simulink model "Charge_2_V1"  (R2017b)
settings: Solver=FixedStepDiscrete  StartTime=0.0  StopTime=1  FixedStep=0.001  RelTol=1e-3
PreLoadFcn:
  | librarySetup
  | eval([bdroot,'_startup']) %Calling [modelName]_startup.m
undefined symbols (not defined in the file or in its folder): A0, A1, Car1__Authorize, Car2_Authorize, CON2, CON3, CON4, Control_Mode_In, CurrentSP, D10, D12, D13, D2, D3, D4, D5, D6, D7, D8, Frequency_High_Point, Frequency_Low_Point, Frequency_Mid_high, Frequency_Mid_low, HVol_High_Point, HVol_Low_Point, HVol_Mid_high, HVol_Mid_low, HVoltage_Factor, SeconCar_ThreePhase, V_Current_five, V_Current_four, V_Current_one, V_Current_six, V_Current_three, V_Current_two, V_Frequency, V_MaxPliot, V_MinPliot, Vol_High_Point, Vol_Low_Point, Vol_Mid_high, Vol_Mid_low, Voltage_Factor, Voltage_Mode_Test
libraries: simulink x331, HANcoder_STM32_Target x30, powerlib_meascontrol x8, simulink_extras x2
(part 2 of 13)

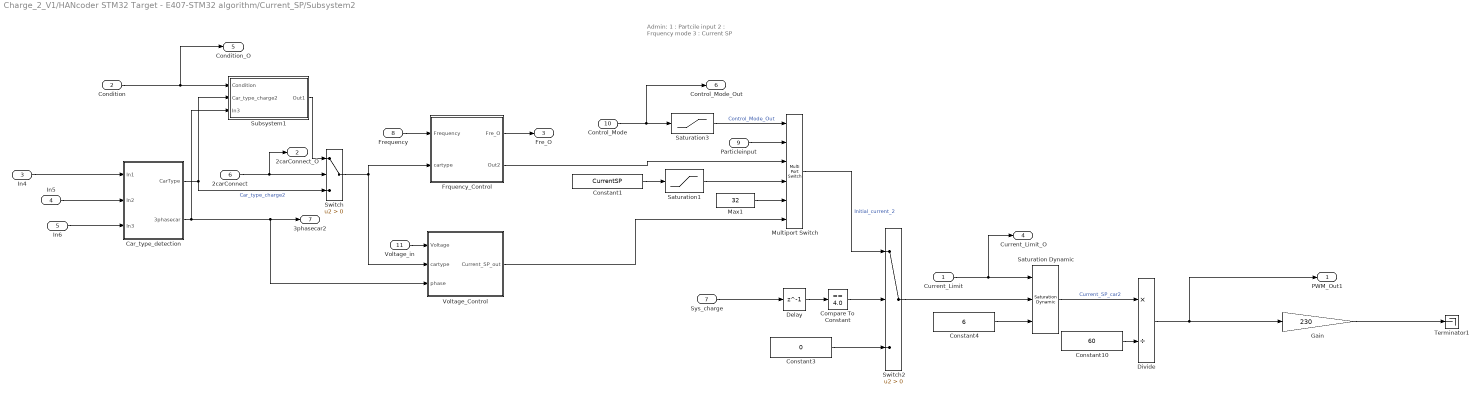
== system Charge_2_V1/HANcoder STM32 Target - E407-STM32 algorithm/Current_SP/Subsystem2 ==
  note: Admin:   1 : Partcile input
      | 		2 : Frquency mode
      | 		3 : Current SP
  Current_Limit : Inport
  Condition : Inport  Port=2
  In4 : Inport  Port=3
  In5 : Inport  Port=4
  In6 : Inport  Port=5
  2carConnect : Inport  Port=6
  Sys_charge : Inport  Port=7
  Frequency : Inport  Port=8
  Particleinput : Inport  Port=9
  Control_Mode : Inport  Port=10
  Voltage_in : Inport  Port=11
  Car_type_detection : Subsystem
  Compare To Constant : simulink/Logic and Bit Operations/Compare To Constant  relop===  const=4.0  OutDataTypeStr=boolean
  Constant1 : Constant  Value=CurrentSP  OutDataTypeStr=single  SampleTime=-1
  Constant10 : Constant  Value=60  OutDataTypeStr=single  SampleTime=-1
  Constant3 : Constant  Value=0  OutDataTypeStr=single  SampleTime=-1
  Constant4 : Constant  Value=6  OutDataTypeStr=single  SampleTime=-1
  Delay : Delay  DelayLength=1  InitialCondition=0
  Divide : Product  Inputs=*/
  Frquency_Control : Subsystem
  Gain : Gain  Gain=230  OutDataTypeStr=single
  Max1 : Constant  Value=32  OutDataTypeStr=single  SampleTime=-1
  Multiport Switch : MultiPortSwitch  Inputs=5
  Saturation Dynamic : simulink/Discontinuities/Saturation Dynamic  OutMin=[]  OutMax=[]  OutDataTypeStr=Inherit: Same as second input  OutDataType=fixdt(1, 16)  OutScaling=2^-10  DoSatur=off
  Saturation1 : Saturate  UpperLimit=32  LowerLimit=6
  Saturation3 : Saturate  UpperLimit=5  LowerLimit=1
  Subsystem1 : Subsystem
  Switch : Switch  Criteria=u2 > Threshold
  Switch2 : Switch  Criteria=u2 > Threshold
  Terminator1 : Terminator
  Voltage_Control : Subsystem
  PWM_Out1 : Outport
  2carConnect_O : Outport  Port=2
  Fre_O : Outport  Port=3
  Current_Limit_O : Outport  Port=4
  Condition_O : Outport  Port=5
  Control_Mode_Out : Outport  Port=6
  3phasecar2 : Outport  Port=7
  wires:
  Compare To Constant/1 -> Switch2/2
  Constant3/1 -> Switch2/3
  Delay/1 -> Compare To Constant/1
  Sys_charge/1 -> Delay/1
  Constant10/1 -> Divide/2
  In5/1 -> Car_type_detection/2(In2)
  Multiport Switch/1 -> Switch2/1  "Initial_current_2"
  In6/1 -> Car_type_detection/3(In3)
  In4/1 -> Car_type_detection/1(In1)
  Constant1/1 -> Saturation1/1
  Car_type_detection/1(CarType) -> Subsystem1/2(Car_type_charge2), Switch/3  "Car_type_charge2"
  Gain/1 -> Terminator1/1
  Divide/1 -> PWM_Out1/1, Gain/1
  Saturation1/1 -> Multiport Switch/4
  Switch2/1 -> Saturation Dynamic/2
  Constant4/1 -> Saturation Dynamic/3
  Current_Limit/1 -> Current_Limit_O/1, Saturation Dynamic/1
  Saturation Dynamic/1 -> Divide/1  "Current_SP_car2"
  Particleinput/1 -> Multiport Switch/2
  Control_Mode/1 -> Control_Mode_Out/1, Saturation3/1
  Saturation3/1 -> Multiport Switch/1  "Control_Mode_Out"
  Max1/1 -> Multiport Switch/5
  Car_type_detection/2(3phasecar) -> Voltage_Control/3(phase), 3phasecar2/1, Subsystem1/3(In3)
  Condition/1 -> Condition_O/1, Subsystem1/1(Condition)
  Subsystem1/1(Out1) -> Switch/1
  2carConnect/1 -> 2carConnect_O/1, Switch/2
  Frequency/1 -> Frquency_Control/1(Frequency)
  Switch/1 -> Voltage_Control/2(cartype), Frquency_Control/2(cartype)
  Frquency_Control/1(Fre_O) -> Fre_O/1
  Frquency_Control/2(Out2) -> Multiport Switch/3
  Voltage_Control/1(Current_SP_out) -> Multiport Switch/6
  Voltage_in/1 -> Voltage_Control/1(Voltage)

== system Charge_2_V1/HANcoder STM32 Target - E407-STM32 algorithm/Current_SP/Voltage_input ==
  In1 : Inport
  In2 : Inport  Port=2
  In3 : Inport  Port=3
  Merge : Merge  Inputs=3
  Signal Conversion : SignalConversion  OverrideOpt=off
  Signal Conversion1 : SignalConversion  OverrideOpt=off
  Signal Conversion2 : SignalConversion  OverrideOpt=off
  Subsystem : Subsystem
  Subsystem3 : Subsystem
  Subsystem4 : Subsystem
  Switch : Switch  Criteria=u2 > Threshold
  Switch1 : Switch  Criteria=u2 > Threshold
  Switch2 : Switch  Criteria=u2 > Threshold
  Out1 : Outport
  wires:
  Switch/1 -> Out1/1
  Subsystem4/1(Out1) -> Switch2/2
  Subsystem/1(Out1) -> Switch/2
  Switch1/1 -> Switch/3
  Subsystem3/1(Out1) -> Switch1/2
  Switch2/1 -> Switch1/3
  Merge/1 -> Switch2/3
  In2/1 -> Signal Conversion2/1, Signal Conversion1/1, Subsystem3/1(In1), Switch1/1, Subsystem/2(In2)
  In3/1 -> Subsystem3/2(In2), Switch2/1, Subsystem4/1(In1)
  In1/1 -> Switch/1, Signal Conversion/1, Subsystem4/2(In2), Subsystem/1(In1)
  Signal Conversion/1 -> Merge/1
  Signal Conversion1/1 -> Merge/2
  Signal Conversion2/1 -> Merge/3

== system Charge_2_V1/HANcoder STM32 Target - E407-STM32 algorithm/Current_SP/Voltage_input1 ==
  In1 : Inport
  In2 : Inport  Port=2
  In3 : Inport  Port=3
  Merge : Merge  Inputs=3
  Signal Conversion : SignalConversion  OverrideOpt=off
  Signal Conversion1 : SignalConversion  OverrideOpt=off
  Signal Conversion2 : SignalConversion  OverrideOpt=off
  Subsystem : Subsystem
  Subsystem3 : Subsystem
  Subsystem4 : Subsystem
  Switch : Switch  Criteria=u2 > Threshold
  Switch1 : Switch  Criteria=u2 > Threshold
  Switch2 : Switch  Criteria=u2 > Threshold
  Out1 : Outport
  wires:
  Merge/1 -> Switch2/3
  Switch2/1 -> Switch1/3
  Subsystem3/1(Out1) -> Switch1/2
  Switch1/1 -> Switch/3
  Subsystem/1(Out1) -> Switch/2
  Subsystem4/1(Out1) -> Switch2/2
  Switch/1 -> Out1/1
  In1/1 -> Subsystem/1(In1), Subsystem4/2(In2), Signal Conversion/1, Switch/1
  In2/1 -> Signal Conversion2/1, Signal Conversion1/1, Subsystem3/1(In1), Switch1/1, Subsystem/2(In2)
  In3/1 -> Subsystem3/2(In2), Switch2/1, Subsystem4/1(In1)
  Signal Conversion/1 -> Merge/1
  Signal Conversion1/1 -> Merge/2
  Signal Conversion2/1 -> Merge/3

== system Charge_2_V1/HANcoder STM32 Target - E407-STM32 algorithm/Energy Meter1/Energy_Meter ==
  Terminator3 : Terminator
  UART init1 : Subsystem  Tag=HANcoder_TARGET_STM32_E407  AncestorBlock=HANcoder_STM32_Target/STM32-E407/UART/UART init  mask(UART init){channel=UART2: CON PD - 8 & 9, baudrate=9600, databits=8, parity=none, stopbits=1, txbufsize=100, rxbufsize=100, useStatusOut=off}
      mask prompts: baudrate "Baudrate (bit/s)"; txbufsize "Transmit buffer size"; rxbufsize "Receive buffer size"; useStatusOut "Use status output"
      mask help:
      | Function
      | ==========
      | Initialized a UART channel.
      |
      | Parameters per channel
      | ======================
      | - Select channel (TX & RX)
      | - Select baudrate
      | - Select number of databits
      | - Select parity
      | - Select number of stopbits
      | - Configure the size of the transmit buffer
      | - Configure the size of the reception buffer
      | - Enable/disable the status output port
      mask init:
      | uartChannelInfoStr = sfcn_uart_init_mcb(2, channel, baudrate, databits, parity, stopbits, txbufsize, rxbufsize, useStatusOut);
      settings: CopyFcn=sfcn_uart_init_chk();  MoveFcn=drawLogos
      mask Help: web('sfcn_uart_init.html')
      mask TypeOptions channel: UART1: CON3 - D1 & D0 | UART2: CON PD - 8 & 9 | UART3: CON PD - 11 & 12 | UART6: UEXT - 3 & 4
      mask Callback channel: sfcn_uart_init_chk();
      mask TypeOptions baudrate: 300 | 600 | 1200 | 2400 | 4800 | 9600 | 19200 | 38400 | 57600 | 115200
      mask TypeOptions databits: 8 | 9
      mask TypeOptions parity: none | even | odd
      mask TypeOptions stopbits: 1 | 2
      mask Display: fprintf('UART init\n%s', uartChannelInfoStr);patch([261 267 267],[8 14 2],[1 0 0]);patch([269 269 275],[14 2 8],[0 0 0.35]);
  UART receive buffer status1 : HANcoder_STM32_Target/STM32-E407/UART/UART receive buffer status  Tag=HANcoder_TARGET_STM32_E407  channel=UART2: CON PD - 8 & 9  tsamp=-1
      settings: SourceProductName=HANcoder STM32 Target
  wires:
  UART receive buffer status1/1 -> Terminator3/1

== system Charge_2_V1/HANcoder STM32 Target - E407-STM32 algorithm/Energy Meter1/Energy_Meter_Recieve ==
  In1 : Inport
  CurrentMeter2 : Subsystem
  Current_Meter : Subsystem
  Fequency : Subsystem
  Subsystem : Subsystem
  Subsystem1 : Subsystem
  Subsystem2 : Subsystem
  Subsystem3 : Subsystem
  Subsystem5 : Subsystem
  Voltage_Meter_1 : Subsystem
  Voltage_Meter_2 : Subsystem
  Current Phase 1 : Outport
  Current phase 2 : Outport  Port=2
  Current phase 3 : Outport  Port=3
  Current phase 4 : Outport  Port=4
  Current phase 5 : Outport  Port=5
  Current phase 6 : Outport  Port=6
  vol1 : Outport  Port=7
  vol2 : Outport  Port=8
  vol3 : Outport  Port=9
  vol4 : Outport  Port=10
  vol5 : Outport  Port=11
  vol6 : Outport  Port=12
  Frequency : Outport  Port=13
  wires:
  In1/1 -> Fequency/1(In1), Voltage_Meter_1/1(In1), Voltage_Meter_2/1(In1), CurrentMeter2/1(In1), Current_Meter/1(In1)
  Subsystem2/1(Out1) -> Subsystem/1(In1), Subsystem1/1(In41)
  Subsystem2/2(Out2) -> Subsystem/2(In3), Subsystem1/2(In1)
  Subsystem2/3(Out3) -> Subsystem/3(In5), Subsystem1/3(In2)
  Subsystem2/4(Out4) -> Subsystem/4(In7), Subsystem1/4(In3)
  Subsystem2/5(Out5) -> Subsystem/5(In9), Subsystem1/5(In4)
  Subsystem2/6(Out6) -> Subsystem/6(In11), Subsystem1/6(In5)
  Subsystem2/7(Out7) -> Subsystem/7(In2), Subsystem1/7(In6)
  Subsystem/1(Current Phase 1) -> Current Phase 1/1
  Subsystem/2(Current phase 2) -> Current phase 2/1
  Subsystem/3(Current phase 3) -> Current phase 3/1
  Subsystem/4(Current phase 4) -> Current phase 4/1
  Subsystem/5(Current phase 5) -> Current phase 5/1
  Subsystem/6(Current phase 6) -> Current phase 6/1
  Subsystem/7(Fre) -> Frequency/1
  Current_Meter/1(Current1) -> Subsystem2/1(In1)
  Current_Meter/2(Current2) -> Subsystem2/2(In2)
  CurrentMeter2/1(byte1) -> Subsystem2/5(In4)
  CurrentMeter2/2(byte6) -> Subsystem2/6(In5)
  CurrentMeter2/3(byte12) -> Subsystem2/7(In6)
  Fequency/1(Fre) -> Subsystem2/9(In8)
  Current_Meter/3(Current3) -> Subsystem2/3(In3)
  Current_Meter/4(check) -> Subsystem2/4(checkID1)
  CurrentMeter2/4(check) -> Subsystem2/8(CheckID2)
  Fequency/2(check) -> Subsystem2/10(CheckID_Fre)
  Voltage_Meter_2/4(check) -> Subsystem3/8(CheckID2)
  Voltage_Meter_2/1(byte5) -> Subsystem3/5(In4)
  Voltage_Meter_2/2(byte9) -> Subsystem3/6(In5)
  Voltage_Meter_2/3(byte13) -> Subsystem3/7(In6)
  Subsystem5/1(Voltage1) -> vol1/1
  Subsystem5/2(Voltage2) -> vol2/1
  Subsystem5/3(Voltage3) -> vol3/1
  Subsystem5/4(Voltage4) -> vol4/1
  Subsystem5/5(Voltage5) -> vol5/1
  Subsystem5/6(Voltage6) -> vol6/1
  Subsystem3/1(Out1) -> Subsystem5/1(In1), Subsystem1/8(In7)
  Subsystem3/2(Out2) -> Subsystem5/2(In3), Subsystem1/9(In8)
  Subsystem3/3(Out3) -> Subsystem5/3(In5), Subsystem1/10(In9)
  Subsystem3/4(Out4) -> Subsystem5/4(In7), Subsystem1/11(In10)
  Subsystem3/5(Out5) -> Subsystem5/5(In9), Subsystem1/12(In11)
  Subsystem3/6(Out6) -> Subsystem5/6(In11), Subsystem1/13(In12)
  Voltage_Meter_1/1(byte5) -> Subsystem3/1(In1)
  Voltage_Meter_1/2(byte9) -> Subsystem3/2(In2)
  Voltage_Meter_1/3(byte13) -> Subsystem3/3(In3)
  Voltage_Meter_1/4(check) -> Subsystem3/4(checkID1)

== system Charge_2_V1/HANcoder STM32 Target - E407-STM32 algorithm/Energy Meter1/Energymeter_Request ==
  Counter Limited1 : simulink/Sources/Counter Limited  uplimit=1400  tsamp=0.001
  "Current_Meter_1 " : Subsystem
  Current_Meter_2 : Subsystem
  Fequency : Subsystem
  "RequestMessages_Enable " : Subsystem
  Voltage_meter_1 : Subsystem
  Voltage_meter_2 : Subsystem
  wires:
  Counter Limited1/1 -> Voltage_meter_1/1(In1), Voltage_meter_2/1(In1), Fequency/1(In1), "RequestMessages_Enable "/1(In1), Current_Meter_2/1(In1), "Current_Meter_1 "/1(In1)

== system Charge_2_V1/HANcoder STM32 Target - E407-STM32 algorithm/Energy Meter1/Particle ==
  Terminator1 : Terminator
  UART init : Subsystem  Tag=HANcoder_TARGET_STM32_E407  AncestorBlock=HANcoder_STM32_Target/STM32-E407/UART/UART init  mask(UART init){channel=UART1: CON3 - D1 & D0, baudrate=9600, databits=8, parity=none, stopbits=1, txbufsize=100, rxbufsize=120, useStatusOut=off}
      mask prompts: baudrate "Baudrate (bit/s)"; txbufsize "Transmit buffer size"; rxbufsize "Receive buffer size"; useStatusOut "Use status output"
      mask help:
      | Function
      | ==========
      | Initialized a UART channel.
      |
      | Parameters per channel
      | ======================
      | - Select channel (TX & RX)
      | - Select baudrate
      | - Select number of databits
      | - Select parity
      | - Select number of stopbits
      | - Configure the size of the transmit buffer
      | - Configure the size of the reception buffer
      | - Enable/disable the status output port
      mask init:
      | uartChannelInfoStr = sfcn_uart_init_mcb(2, channel, baudrate, databits, parity, stopbits, txbufsize, rxbufsize, useStatusOut);
      settings: CopyFcn=sfcn_uart_init_chk();  MoveFcn=drawLogos
      mask Help: web('sfcn_uart_init.html')
      mask TypeOptions channel: UART1: CON3 - D1 & D0 | UART2: CON PD - 8 & 9 | UART3: CON PD - 11 & 12 | UART6: UEXT - 3 & 4
      mask Callback channel: sfcn_uart_init_chk();
      mask TypeOptions baudrate: 300 | 600 | 1200 | 2400 | 4800 | 9600 | 19200 | 38400 | 57600 | 115200
      mask TypeOptions databits: 8 | 9
      mask TypeOptions parity: none | even | odd
      mask TypeOptions stopbits: 1 | 2
      mask Display: fprintf('UART init\n%s', uartChannelInfoStr);patch([261 267 267],[8 14 2],[1 0 0]);patch([269 269 275],[14 2 8],[0 0 0.35]);
  UART receive buffer status : HANcoder_STM32_Target/STM32-E407/UART/UART receive buffer status  Tag=HANcoder_TARGET_STM32_E407  channel=UART1: CON3 - D1 & D0  tsamp=-1
      settings: SourceProductName=HANcoder STM32 Target
  wires:
  UART receive buffer status/1 -> Terminator1/1  "Status"

== system Charge_2_V1/HANcoder STM32 Target - E407-STM32 algorithm/Partclie_SP_Receive/SP1 ==
  In1 : Inport
  Compare To Constant : simulink/Logic and Bit Operations/Compare To Constant  relop===  const=1  OutDataTypeStr=uint8
  Compare To Constant1 : simulink/Logic and Bit Operations/Compare To Constant  relop===  const=2  OutDataTypeStr=uint8
  Compare To Constant2 : simulink/Logic and Bit Operations/Compare To Constant  relop===  const=3  OutDataTypeStr=uint8
  Compare To Constant3 : simulink/Logic and Bit Operations/Compare To Constant  relop===  const=4  OutDataTypeStr=uint8
  Compare To Constant4 : simulink/Logic and Bit Operations/Compare To Constant  relop===  const=2.0  OutDataTypeStr=boolean
  Compare To Constant5 : simulink/Logic and Bit Operations/Compare To Constant  relop===  const=254.0  OutDataTypeStr=boolean
  Compare To Constant6 : simulink/Logic and Bit Operations/Compare To Constant  relop===  const=1.0  OutDataTypeStr=boolean
  Compare To Constant7 : simulink/Logic and Bit Operations/Compare To Constant  relop=>=  const=6.0  OutDataTypeStr=boolean
  Compare To Constant8 : simulink/Logic and Bit Operations/Compare To Constant  relop===  const=255.0  OutDataTypeStr=boolean
  Read_Gyro : Subsystem  TreatAsAtomicUnit=on
  Read_Gyro1 : Subsystem  TreatAsAtomicUnit=on
  Read_Gyro2 : Subsystem  TreatAsAtomicUnit=on
  Read_Gyro3 : Subsystem  TreatAsAtomicUnit=on
  Subsystem : Subsystem
  Out1 : Outport
  Out2 : Outport  Port=2
  wires:
  Compare To Constant2/1 -> Read_Gyro2/Trigger
  Compare To Constant3/1 -> Read_Gyro3/Trigger
  In1/1 -> Compare To Constant3/1, Compare To Constant2/1, Compare To Constant/1, Compare To Constant1/1
  Compare To Constant1/1 -> Read_Gyro1/Trigger
  Read_Gyro1/1(Out1) -> Compare To Constant4/1, Compare To Constant6/1  "SP_ID"
  Read_Gyro/1(Out1) -> Compare To Constant5/1  "Setpoin_check1"
  Compare To Constant/1 -> Read_Gyro/Trigger
  Read_Gyro3/1(Out1) -> Compare To Constant8/1  "End_SP1"
  Read_Gyro2/1(Out1) -> Subsystem/4(Setpoint1), Compare To Constant7/1  "Setpoint1"
  Compare To Constant5/1 -> Subsystem/1(In1)
  Compare To Constant6/1 -> Subsystem/2(In2)
  Compare To Constant4/1 -> Subsystem/3(In3)
  Compare To Constant7/1 -> Subsystem/5(In5)
  Compare To Constant8/1 -> Subsystem/6(In6)
  Subsystem/1(SP1_P) -> Out1/1
  Subsystem/2(SP2_P) -> Out2/1

== system Charge_2_V1/HANcoder STM32 Target - E407-STM32 algorithm/Car1/PWM/PWM Init ==
  S-Function : S-Function  FunctionName=sfcn_pwmout_init  SFunctionDeploymentMode=off  EnableBusSupport=off
  Term1 : Terminator
  wires:
  S-Function/1 -> Term1/1

== system Charge_2_V1/HANcoder STM32 Target - E407-STM32 algorithm/Car1/Pilotcar1/MVA_Filter ==
  In1 : Inport
  Add2 : Sum  Inputs=++++++++++
  Delay1 : Delay  InitialCondition=0
  Delay2 : Delay  DelayLength=1  InitialCondition=0
  Delay3 : Delay  DelayLength=3  InitialCondition=0
  Delay4 : Delay  DelayLength=4  InitialCondition=0
  Delay5 : Delay  DelayLength=5  InitialCondition=0
  Delay6 : Delay  DelayLength=6  InitialCondition=0
  Delay7 : Delay  DelayLength=7  InitialCondition=0
  Delay8 : Delay  DelayLength=8  InitialCondition=0
  Delay9 : Delay  DelayLength=9  InitialCondition=0
  Gain3 : Gain  Gain=1/2
  Out1 : Outport
  wires:
  Add2/1 -> Gain3/1
  In1/1 -> Delay9/1, Delay8/1, Delay7/1, Delay6/1, Delay5/1, Delay4/1, Delay3/1, Delay1/1, Delay2/1, Add2/1
  Delay2/1 -> Add2/2
  Gain3/1 -> Out1/1

== system Charge_2_V1/HANcoder STM32 Target - E407-STM32 algorithm/Car1/Pilotcar1/Max_filter ==
  In1 : Inport
  If : If  IfExpression=u1 < 0
  If Action Subsystem : Subsystem  TreatAsAtomicUnit=on
  If Action Subsystem1 : Subsystem  TreatAsAtomicUnit=on
  Merge : Merge
  Unit Delay : UnitDelay  SampleTime=-1
  Out1 : Outport
  wires:
  Merge/1 -> Unit Delay/1, Out1/1
  If Action Subsystem1/1(Out1) -> Merge/2
  Unit Delay/1 -> If Action Subsystem/1(In1)
  If/2 -> If Action Subsystem1/Action
  In1/1 -> If/1, If Action Subsystem1/1(In1)
  If/1 -> If Action Subsystem/Action
  If Action Subsystem/1(Out1) -> Merge/1

== system Charge_2_V1/HANcoder STM32 Target - E407-STM32 algorithm/Car1/Pilotcar1/Min_filter ==
  In1 : Inport
  If Action Subsystem2 : Subsystem  TreatAsAtomicUnit=on
  If Action Subsystem3 : Subsystem  TreatAsAtomicUnit=on
  If1 : If  IfExpression=u1 >= 0
  Merge1 : Merge
  Unit Delay1 : UnitDelay  SampleTime=-1
  Out1 : Outport
  wires:
  Merge1/1 -> Out1/1, Unit Delay1/1
  In1/1 -> If Action Subsystem3/1(In1), If1/1
  If Action Subsystem2/1(Out1) -> Merge1/1
  If1/1 -> If Action Subsystem2/Action
  If1/2 -> If Action Subsystem3/Action
  Unit Delay1/1 -> If Action Subsystem2/1(In1)
  If Action Subsystem3/1(Out1) -> Merge1/2

== system Charge_2_V1/HANcoder STM32 Target - E407-STM32 algorithm/Car2/PWM/PWM Init ==
  S-Function : S-Function  FunctionName=sfcn_pwmout_init  SFunctionDeploymentMode=off  EnableBusSupport=off
  Term1 : Terminator
  wires:
  S-Function/1 -> Term1/1

== system Charge_2_V1/HANcoder STM32 Target - E407-STM32 algorithm/Car2/Pilotcar2/MVA_Filter ==
  In1 : Inport
  Add2 : Sum  Inputs=++++++++++
  Delay1 : Delay  InitialCondition=0
  Delay2 : Delay  DelayLength=1  InitialCondition=0
  Delay3 : Delay  DelayLength=3  InitialCondition=0
  Delay4 : Delay  DelayLength=4  InitialCondition=0
  Delay5 : Delay  DelayLength=5  InitialCondition=0
  Delay6 : Delay  DelayLength=6  InitialCondition=0
  Delay7 : Delay  DelayLength=7  InitialCondition=0
  Delay8 : Delay  DelayLength=8  InitialCondition=0
  Delay9 : Delay  DelayLength=9  InitialCondition=0
  Gain3 : Gain  Gain=1/2
  Out1 : Outport
  wires:
  Gain3/1 -> Out1/1
  Delay2/1 -> Add2/2
  In1/1 -> Add2/1, Delay2/1, Delay1/1, Delay3/1, Delay4/1, Delay5/1, Delay6/1, Delay7/1, Delay8/1, Delay9/1
  Add2/1 -> Gain3/1

== system Charge_2_V1/HANcoder STM32 Target - E407-STM32 algorithm/Car2/Pilotcar2/Max_filter ==
  In1 : Inport
  If : If  IfExpression=u1 < 0
  If Action Subsystem : Subsystem  TreatAsAtomicUnit=on
  If Action Subsystem1 : Subsystem  TreatAsAtomicUnit=on
  Merge : Merge
  Unit Delay : UnitDelay  SampleTime=-1
  Out1 : Outport
  wires:
  If Action Subsystem/1(Out1) -> Merge/1
  If/1 -> If Action Subsystem/Action
  In1/1 -> If Action Subsystem1/1(In1), If/1
  If/2 -> If Action Subsystem1/Action
  Unit Delay/1 -> If Action Subsystem/1(In1)
  If Action Subsystem1/1(Out1) -> Merge/2
  Merge/1 -> Out1/1, Unit Delay/1

== system Charge_2_V1/HANcoder STM32 Target - E407-STM32 algorithm/Car2/Pilotcar2/Min_filter ==
  In1 : Inport
  If Action Subsystem2 : Subsystem  TreatAsAtomicUnit=on
  If Action Subsystem3 : Subsystem  TreatAsAtomicUnit=on
  If1 : If  IfExpression=u1 >= 0
  Merge1 : Merge
  Unit Delay1 : UnitDelay  SampleTime=-1
  Out1 : Outport
  wires:
  If Action Subsystem3/1(Out1) -> Merge1/2
  Unit Delay1/1 -> If Action Subsystem2/1(In1)
  If1/2 -> If Action Subsystem3/Action
  If1/1 -> If Action Subsystem2/Action
  If Action Subsystem2/1(Out1) -> Merge1/1
  In1/1 -> If1/1, If Action Subsystem3/1(In1)
  Merge1/1 -> Unit Delay1/1, Out1/1

== system Charge_2_V1/HANcoder STM32 Target - E407-STM32 algorithm/Current_SP/Subsystem1/Car_type_detection ==
  note: 1 means 3 phase, 0 means 1phase
  note: 1 mean 32A, 0 ,mean 16A
  In1 : Inport
  In2 : Inport  Port=2
  In3 : Inport  Port=3
  Bitwise Operator : simulink/Logic and Bit Operations/Bitwise Operator  logicop=AND  UseBitMask=off  NumInputPorts=2  BitMask=bin2dec('11011001')  BitMaskRealWorld=Stored Integer
  Car_type_detection2 : simulink/Logic and Bit Operations/Compare To Constant  relop=>  const=18.0  OutDataTypeStr=boolean
  Car_type_detection3 : simulink/Logic and Bit Operations/Compare To Constant  relop=>  const=18.0  OutDataTypeStr=boolean
  Car_type_detection4 : simulink/Logic and Bit Operations/Compare To Constant  relop=>  const=18.0  OutDataTypeStr=boolean
  Car_type_detection5 : simulink/Logic and Bit Operations/Compare To Constant  relop=>  const=6.0  OutDataTypeStr=boolean
  Car_type_detection6 : simulink/Logic and Bit Operations/Compare To Constant  relop=>  const=6.0  OutDataTypeStr=boolean
  Car_type_detection7 : simulink/Logic and Bit Operations/Compare To Constant  relop=>  const=6.0  OutDataTypeStr=boolean
  Constant3 : Constant  OutDataTypeStr=boolean  SampleTime=-1
  Data Type Conversion : DataTypeConversion  OutDataTypeStr=double
  Logical Operator : Logic  Operator=OR  Inputs=3  AllPortsSameDT=off  OutDataTypeStr=boolean
  Logical Operator1 : Logic  Inputs=3  AllPortsSameDT=off  OutDataTypeStr=boolean
  Logical Operator2 : Logic  Operator=NOT  AllPortsSameDT=off  OutDataTypeStr=boolean
  S-R Flip-Flop : simulink_extras/Flip Flops/S-R Flip-Flop  initial_condition=0
  Terminator : Terminator
  Terminator1 : Terminator
  CarType : Outport  SampleTime=0.1
  3phasecar2 : Outport  Port=2  SampleTime=0.1
  wires:
  In2/1 -> Car_type_detection3/1, Car_type_detection6/1
  In1/1 -> Car_type_detection2/1, Car_type_detection5/1
  In3/1 -> Car_type_detection4/1, Car_type_detection7/1
  Logical Operator/1 -> Bitwise Operator/1
  S-R Flip-Flop/1 -> Data Type Conversion/1
  S-R Flip-Flop/2 -> Terminator/1
  Logical Operator2/1 -> S-R Flip-Flop/2
  Constant3/1 -> Bitwise Operator/2
  Bitwise Operator/1 -> Logical Operator2/1, S-R Flip-Flop/1
  Logical Operator1/1 -> 3phasecar2/1, Terminator1/1
  Data Type Conversion/1 -> CarType/1
  Car_type_detection2/1 -> Logical Operator/1
  Car_type_detection3/1 -> Logical Operator/2
  Car_type_detection4/1 -> Logical Operator/3
  Car_type_detection5/1 -> Logical Operator1/1
  Car_type_detection6/1 -> Logical Operator1/2
  Car_type_detection7/1 -> Logical Operator1/3

== system Charge_2_V1/HANcoder STM32 Target - E407-STM32 algorithm/Current_SP/Subsystem1/Fre_Control ==
  Frequency : Inport
  In2 : Inport  Port=2
  16A_Car : Subsystem
  32A_Car1 : Subsystem
  Bus Creator : BusCreator  Inputs=3
  Bus Creator1 : BusCreator  Inputs=3
  Bus Selector : BusSelector  OutputSignals=signal1,signal2,signal3
  Saturation2 : Saturate  UpperLimit=32  LowerLimit=6
  Subsystem1 : Subsystem
  Switch1 : Switch  Criteria=u2 > Threshold
  Out1 : Outport
  wires:
  32A_Car1/1(Out1) -> Bus Creator1/1
  Subsystem1/1(Out1) -> Saturation2/1
  Bus Creator/1 -> Switch1/3
  Bus Selector/1 -> Subsystem1/2(In2)  "<signal1>"
  Switch1/1 -> Bus Selector/1
  32A_Car1/2(Out2) -> Bus Creator1/2
  Saturation2/1 -> Out1/1
  In2/1 -> Switch1/2
  16A_Car/2(Out2) -> Bus Creator/2
  32A_Car1/3(Out3) -> Bus Creator1/3
  Bus Creator1/1 -> Switch1/1
  16A_Car/3(Out3) -> Bus Creator/3
  16A_Car/1(Out1) -> Bus Creator/1
  Bus Selector/3 -> Subsystem1/4(In4)  "<signal3>"
  Frequency/1 -> Subsystem1/1(In1), 16A_Car/1(Fre), 32A_Car1/1(fre)
  Bus Selector/2 -> Subsystem1/3(In3)  "<signal2>"

== system Charge_2_V1/HANcoder STM32 Target - E407-STM32 algorithm/Current_SP/Subsystem1/Subsystem2 ==
  Condition : Inport
  Car_type_charge2 : Inport  Port=2
  In4 : Inport  Port=3
  Logical Operator : Logic  Inputs=3  AllPortsSameDT=off  OutDataTypeStr=boolean
  Logical Operator2 : Logic  Operator=NOT  AllPortsSameDT=off  OutDataTypeStr=boolean
  Out1 : Outport
  wires:
  In4/1 -> Logical Operator2/1
  Car_type_charge2/1 -> Logical Operator/3
  Condition/1 -> Logical Operator/1
  Logical Operator/1 -> Out1/1
  Logical Operator2/1 -> Logical Operator/2

== system Charge_2_V1/HANcoder STM32 Target - E407-STM32 algorithm/Current_SP/Subsystem1/Voltage_Control ==
  Voltage : Inport
  cartype : Inport  Port=2
  phase : Inport  Port=3
  1phase : Subsystem
  3phase : Subsystem
  Compare To Constant : simulink/Logic and Bit Operations/Compare To Constant  relop=>  const=320  OutDataTypeStr=boolean
  Compare To Constant1 : simulink/Logic and Bit Operations/Compare To Constant  relop=<  const=320  OutDataTypeStr=boolean
  Constant : Constant  Value=3  SampleTime=-1
  Data Type Conversion : DataTypeConversion  OutDataTypeStr=single
  Product : Product
  Sqrt : Sqrt  SaturateOnIntegerOverflow=on
  Switch1 : Switch  Criteria=u2 > Threshold
  Switch2 : Switch  Criteria=u2 > Threshold
  Current_SP_out : Outport
  wires:
  Constant/1 -> Sqrt/1
  Voltage/1 -> Product/2, Switch2/3
  phase/1 -> Switch1/2, Switch2/2
  Sqrt/1 -> Product/1
  Product/1 -> Switch2/1
  Switch2/1 -> 1phase/1(Vol), Compare To Constant1/1, Compare To Constant/1, 3phase/1(Vol)
  Compare To Constant/1 -> 3phase/Trigger
  Compare To Constant1/1 -> 1phase/Trigger
  cartype/1 -> 1phase/2(cartype), 3phase/2(cartype)
  Switch1/1 -> Data Type Conversion/1
  3phase/1(Out1) -> Switch1/1
  1phase/1(Out1) -> Switch1/3
  Data Type Conversion/1 -> Current_SP_out/1

== system Charge_2_V1/HANcoder STM32 Target - E407-STM32 algorithm/Current_SP/Subsystem2/Car_type_detection ==
  note: 1 means 3phase 0 means 1 phase
  note: 1 mean 32A, 0 ,mean 16 A
  In1 : Inport
  In2 : Inport  Port=2
  In3 : Inport  Port=3
  Bitwise Operator : simulink/Logic and Bit Operations/Bitwise Operator  logicop=AND  UseBitMask=off  NumInputPorts=2  BitMask=bin2dec('11011001')  BitMaskRealWorld=Stored Integer
  Car_type_detection3 : simulink/Logic and Bit Operations/Compare To Constant  relop=>  const=18.0  OutDataTypeStr=boolean
  Car_type_detection4 : simulink/Logic and Bit Operations/Compare To Constant  relop=>  const=18.0  OutDataTypeStr=boolean
  Car_type_detection5 : simulink/Logic and Bit Operations/Compare To Constant  relop=>  const=6.0  OutDataTypeStr=boolean
  Car_type_detection6 : simulink/Logic and Bit Operations/Compare To Constant  relop=>  const=6.0  OutDataTypeStr=boolean
  Car_type_detection7 : simulink/Logic and Bit Operations/Compare To Constant  relop=>  const=6.0  OutDataTypeStr=boolean
  Constant3 : Constant  OutDataTypeStr=boolean  SampleTime=-1
  Data Type Conversion : DataTypeConversion  OutDataTypeStr=double
  Logical Operator : Logic  Operator=OR  Inputs=3  AllPortsSameDT=off  OutDataTypeStr=boolean
  Logical Operator1 : Logic  Inputs=3  AllPortsSameDT=off  OutDataTypeStr=boolean
  Logical Operator2 : Logic  Operator=NOT  AllPortsSameDT=off  OutDataTypeStr=boolean
  S-R Flip-Flop : simulink_extras/Flip Flops/S-R Flip-Flop  initial_condition=0
  Terminator : Terminator
  Terminator1 : Terminator
  n2 : simulink/Logic and Bit Operations/Compare To Constant  relop=>  const=18.0  OutDataTypeStr=boolean
  CarType : Outport
  3phasecar : Outport  Port=2
  wires:
  Bitwise Operator/1 -> Logical Operator2/1, S-R Flip-Flop/1
  Constant3/1 -> Bitwise Operator/2
  S-R Flip-Flop/2 -> Terminator/1
  S-R Flip-Flop/1 -> Data Type Conversion/1
  Logical Operator/1 -> Bitwise Operator/1
  In3/1 -> Car_type_detection4/1, Car_type_detection7/1
  In1/1 -> n2/1, Car_type_detection5/1
  In2/1 -> Car_type_detection3/1, Car_type_detection6/1
  Logical Operator1/1 -> Terminator1/1, 3phasecar/1
  Logical Operator2/1 -> S-R Flip-Flop/2
  Data Type Conversion/1 -> CarType/1
  n2/1 -> Logical Operator/1
  Car_type_detection3/1 -> Logical Operator/2
  Car_type_detection4/1 -> Logical Operator/3
  Car_type_detection5/1 -> Logical Operator1/1
  Car_type_detection6/1 -> Logical Operator1/2
  Car_type_detection7/1 -> Logical Operator1/3

== system Charge_2_V1/HANcoder STM32 Target - E407-STM32 algorithm/Current_SP/Subsystem2/Frquency_Control ==
  Frequency : Inport
  cartype : Inport  Port=2
  16A_Car : Subsystem
  32A_Car : Subsystem
  Bus Creator : BusCreator  Inputs=3
  Bus Creator1 : BusCreator  Inputs=3
  Bus Selector : BusSelector  OutputSignals=signal1,signal2,signal3
  Saturation2 : Saturate  UpperLimit=32  LowerLimit=6
  Subsystem : Subsystem
  Switch1 : Switch  Criteria=u2 > Threshold
  Fre_O : Outport
  Out2 : Outport  Port=2
  wires:
  Bus Creator1/1 -> Switch1/1
  Bus Selector/3 -> Subsystem/4(In4)  "<signal3>"
  Saturation2/1 -> Out2/1
  Bus Selector/2 -> Subsystem/3(In3)  "<signal2>"
  16A_Car/3(Out3) -> Bus Creator/3
  32A_Car/3(Out3) -> Bus Creator1/3
  32A_Car/1(Out1) -> Bus Creator1/1
  16A_Car/2(Out2) -> Bus Creator/2
  Frequency/1 -> 32A_Car/1(fre), 16A_Car/1(Fre), Fre_O/1, Subsystem/1(In1)
  16A_Car/1(Out1) -> Bus Creator/1
  32A_Car/2(Out2) -> Bus Creator1/2
  Bus Selector/1 -> Subsystem/2(In2)  "<signal1>"
  Switch1/1 -> Bus Selector/1
  cartype/1 -> Switch1/2
  Subsystem/1(Out1) -> Saturation2/1
  Bus Creator/1 -> Switch1/3

== system Charge_2_V1/HANcoder STM32 Target - E407-STM32 algorithm/Current_SP/Subsystem2/Subsystem1 ==
  Condition : Inport
  Car_type_charge2 : Inport  Port=2
  In3 : Inport  Port=3
  Logical Operator : Logic  Inputs=3  AllPortsSameDT=off  OutDataTypeStr=boolean
  Logical Operator2 : Logic  Operator=NOT  AllPortsSameDT=off  OutDataTypeStr=boolean
  Out1 : Outport
  wires:
  In3/1 -> Logical Operator2/1
  Car_type_charge2/1 -> Logical Operator/3
  Condition/1 -> Logical Operator/1
  Logical Operator/1 -> Out1/1
  Logical Operator2/1 -> Logical Operator/2

== system Charge_2_V1/HANcoder STM32 Target - E407-STM32 algorithm/Current_SP/Subsystem2/Voltage_Control ==
  Voltage : Inport
  cartype : Inport  Port=2
  phase : Inport  Port=3
  1phase : Subsystem
  3phase : Subsystem
  Compare To Constant : simulink/Logic and Bit Operations/Compare To Constant  relop=>  const=320  OutDataTypeStr=boolean
  Compare To Constant1 : simulink/Logic and Bit Operations/Compare To Constant  relop=<  const=320  OutDataTypeStr=boolean
  Constant : Constant  Value=3  OutDataTypeStr=single  SampleTime=-1
  Data Type Conversion : DataTypeConversion  OutDataTypeStr=single
  Product : Product
  Sqrt : Sqrt  SaturateOnIntegerOverflow=on
  Switch1 : Switch  Criteria=u2 > Threshold
  Switch2 : Switch  Criteria=u2 > Threshold
  Current_SP_out : Outport
  wires:
  Constant/1 -> Sqrt/1
  Voltage/1 -> Product/2, Switch2/3
  phase/1 -> Switch1/2, Switch2/2
  Sqrt/1 -> Product/1
  Product/1 -> Switch2/1
  Switch2/1 -> Compare To Constant/1, 3phase/1(Vol), 1phase/1(Vol), Compare To Constant1/1  "voltage_de"
  Compare To Constant/1 -> 3phase/Trigger
  Compare To Constant1/1 -> 1phase/Trigger
  cartype/1 -> 1phase/2(cartype), 3phase/2(cartype)
  Switch1/1 -> Data Type Conversion/1
  3phase/1(Out1) -> Switch1/1  "VoltageControl3phaseout"
  1phase/1(Out1) -> Switch1/3  "VoltageControl1phaseout"
  Data Type Conversion/1 -> Current_SP_out/1

== system Charge_2_V1/HANcoder STM32 Target - E407-STM32 algorithm/Current_SP/Voltage_input/Subsystem ==
  In1 : Inport
  In2 : Inport  Port=2
  Add : Sum  Inputs=+-
  Vol_Chang : Subsystem
  Out1 : Outport
  wires:
  In1/1 -> Add/1
  Vol_Chang/1(Out1) -> Out1/1
  Add/1 -> Vol_Chang/1(In1)
  In2/1 -> Add/2

== system Charge_2_V1/HANcoder STM32 Target - E407-STM32 algorithm/Current_SP/Voltage_input/Subsystem3 ==
  In1 : Inport
  In2 : Inport  Port=2
  Add : Sum  Inputs=+-
  Vol_Chang : Subsystem
  Out1 : Outport
  wires:
  In2/1 -> Add/2
  Add/1 -> Vol_Chang/1(In1)
  Vol_Chang/1(Out1) -> Out1/1
  In1/1 -> Add/1

== system Charge_2_V1/HANcoder STM32 Target - E407-STM32 algorithm/Current_SP/Voltage_input/Subsystem4 ==
  In1 : Inport
  In2 : Inport  Port=2
  Add : Sum  Inputs=+-
  Vol_Chang : Subsystem
  Out1 : Outport
  wires:
  In1/1 -> Add/1
  Vol_Chang/1(Out1) -> Out1/1
  Add/1 -> Vol_Chang/1(In1)
  In2/1 -> Add/2

== system Charge_2_V1/HANcoder STM32 Target - E407-STM32 algorithm/Current_SP/Voltage_input1/Subsystem ==
  In1 : Inport
  In2 : Inport  Port=2
  Add : Sum  Inputs=+-
  Vol_Chang : Subsystem
  Out1 : Outport
  wires:
  In2/1 -> Add/2
  Add/1 -> Vol_Chang/1(In1)
  Vol_Chang/1(Out1) -> Out1/1
  In1/1 -> Add/1

== system Charge_2_V1/HANcoder STM32 Target - E407-STM32 algorithm/Current_SP/Voltage_input1/Subsystem3 ==
  In1 : Inport
  In2 : Inport  Port=2
  Add : Sum  Inputs=+-
  Vol_Chang : Subsystem
  Out1 : Outport
  wires:
  In1/1 -> Add/1
  Vol_Chang/1(Out1) -> Out1/1
  Add/1 -> Vol_Chang/1(In1)
  In2/1 -> Add/2

== system Charge_2_V1/HANcoder STM32 Target - E407-STM32 algorithm/Current_SP/Voltage_input1/Subsystem4 ==
  In1 : Inport
  In2 : Inport  Port=2
  Add : Sum  Inputs=+-
  Vol_Chang : Subsystem
  Out1 : Outport
  wires:
  In2/1 -> Add/2
  Add/1 -> Vol_Chang/1(In1)
  Vol_Chang/1(Out1) -> Out1/1
  In1/1 -> Add/1

== system Charge_2_V1/HANcoder STM32 Target - E407-STM32 algorithm/Energy Meter1/Energy_Meter/UART init1 ==
  Level-2 M-file S-Function : M-S-Function  FunctionName=sfcn_uart_init
  Term1 : Terminator
  wires:
  Level-2 M-file S-Function/1 -> Term1/1

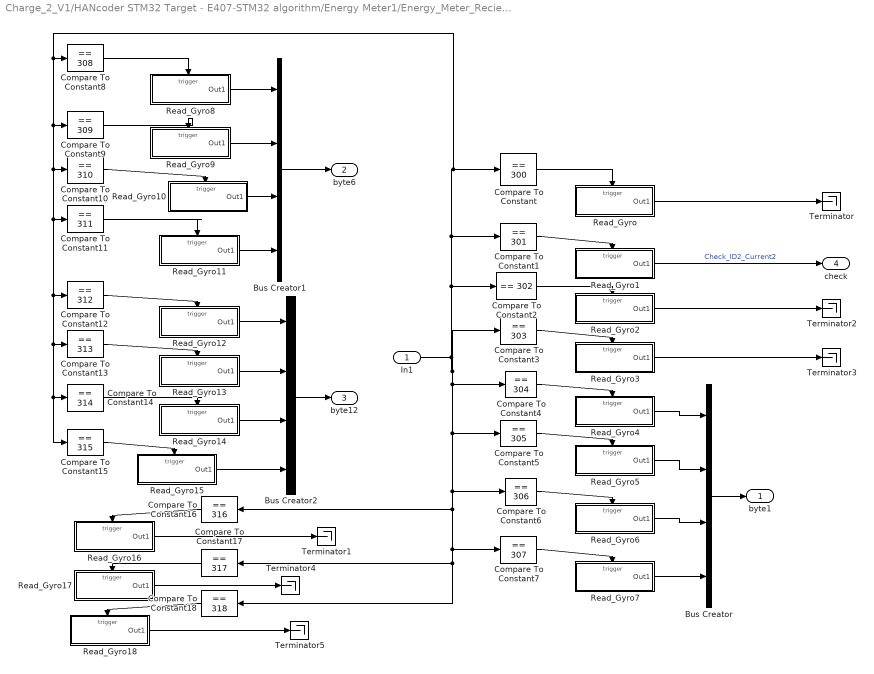
== system Charge_2_V1/HANcoder STM32 Target - E407-STM32 algorithm/Energy Meter1/Energy_Meter_Recieve/CurrentMeter2 ==
  In1 : Inport
  Bus Creator : BusCreator  Inputs=4
  Bus Creator1 : BusCreator  Inputs=4
  Bus Creator2 : BusCreator  Inputs=4
  Compare To Constant : simulink/Logic and Bit Operations/Compare To Constant  relop===  const=300  OutDataTypeStr=uint8
  Compare To Constant1 : simulink/Logic and Bit Operations/Compare To Constant  relop===  const=301  OutDataTypeStr=uint8
  Compare To Constant10 : simulink/Logic and Bit Operations/Compare To Constant  relop===  const=310  OutDataTypeStr=uint8
  Compare To Constant11 : simulink/Logic and Bit Operations/Compare To Constant  relop===  const=311  OutDataTypeStr=uint8
  Compare To Constant12 : simulink/Logic and Bit Operations/Compare To Constant  relop===  const=312  OutDataTypeStr=uint8
  Compare To Constant13 : simulink/Logic and Bit Operations/Compare To Constant  relop===  const=313  OutDataTypeStr=uint8
  Compare To Constant14 : simulink/Logic and Bit Operations/Compare To Constant  relop===  const=314  OutDataTypeStr=uint8
  Compare To Constant15 : simulink/Logic and Bit Operations/Compare To Constant  relop===  const=315  OutDataTypeStr=uint8
  Compare To Constant16 : simulink/Logic and Bit Operations/Compare To Constant  relop===  const=316  OutDataTypeStr=uint8
  Compare To Constant17 : simulink/Logic and Bit Operations/Compare To Constant  relop===  const=317  OutDataTypeStr=uint8
  Compare To Constant18 : simulink/Logic and Bit Operations/Compare To Constant  relop===  const=318  OutDataTypeStr=uint8
  Compare To Constant2 : simulink/Logic and Bit Operations/Compare To Constant  relop===  const=302  OutDataTypeStr=uint8
  Compare To Constant3 : simulink/Logic and Bit Operations/Compare To Constant  relop===  const=303  OutDataTypeStr=uint8
  Compare To Constant4 : simulink/Logic and Bit Operations/Compare To Constant  relop===  const=304  OutDataTypeStr=uint8
  Compare To Constant5 : simulink/Logic and Bit Operations/Compare To Constant  relop===  const=305  OutDataTypeStr=uint8
  Compare To Constant6 : simulink/Logic and Bit Operations/Compare To Constant  relop===  const=306  OutDataTypeStr=uint8
  Compare To Constant7 : simulink/Logic and Bit Operations/Compare To Constant  relop===  const=307  OutDataTypeStr=uint8
  Compare To Constant8 : simulink/Logic and Bit Operations/Compare To Constant  relop===  const=308  OutDataTypeStr=uint8
  Compare To Constant9 : simulink/Logic and Bit Operations/Compare To Constant  relop===  const=309  OutDataTypeStr=uint8
  Read_Gyro : Subsystem  TreatAsAtomicUnit=on
  Read_Gyro1 : Subsystem  TreatAsAtomicUnit=on
  Read_Gyro10 : Subsystem  TreatAsAtomicUnit=on
  Read_Gyro11 : Subsystem  TreatAsAtomicUnit=on
  Read_Gyro12 : Subsystem  TreatAsAtomicUnit=on
  Read_Gyro13 : Subsystem  TreatAsAtomicUnit=on
  Read_Gyro14 : Subsystem  TreatAsAtomicUnit=on
  Read_Gyro15 : Subsystem  TreatAsAtomicUnit=on
  Read_Gyro16 : Subsystem  TreatAsAtomicUnit=on
  Read_Gyro17 : Subsystem  TreatAsAtomicUnit=on
  Read_Gyro18 : Subsystem  TreatAsAtomicUnit=on
  Read_Gyro2 : Subsystem  TreatAsAtomicUnit=on
  Read_Gyro3 : Subsystem  TreatAsAtomicUnit=on
  Read_Gyro4 : Subsystem  TreatAsAtomicUnit=on
  Read_Gyro5 : Subsystem  TreatAsAtomicUnit=on
  Read_Gyro6 : Subsystem  TreatAsAtomicUnit=on
  Read_Gyro7 : Subsystem  TreatAsAtomicUnit=on
  Read_Gyro8 : Subsystem  TreatAsAtomicUnit=on
  Read_Gyro9 : Subsystem  TreatAsAtomicUnit=on
  Terminator{,1..5} (6 alike) : Terminator
  byte1 : Outport
  byte6 : Outport  Port=2
  byte12 : Outport  Port=3
  check : Outport  Port=4
  wires:
  Read_Gyro18/1(Out1) -> Terminator5/1
  Read_Gyro17/1(Out1) -> Terminator4/1
  Compare To Constant18/1 -> Read_Gyro18/Trigger
  Compare To Constant17/1 -> Read_Gyro17/Trigger
  Compare To Constant16/1 -> Read_Gyro16/Trigger
  Compare To Constant15/1 -> Read_Gyro15/Trigger
  Compare To Constant14/1 -> Read_Gyro14/Trigger
  Compare To Constant8/1 -> Read_Gyro8/Trigger
  In1/1 -> Compare To Constant3/1, Compare To Constant4/1, Compare To Constant5/1, Compare To Constant6/1, Compare To Constant16/1, Compare To Constant7/1, Compare To Constant18/1, Compare To Constant17/1, Compare To Constant2/1, Compare To Constant1/1, Compare To Constant15/1, Compare To Constant14/1, Compare To Constant13/1, Compare To Constant12/1, Compare To Constant11/1, Compare To Constant10/1, Compare To Constant9/1, Compare To Constant8/1, Compare To Constant/1
  Compare To Constant13/1 -> Read_Gyro13/Trigger
  Compare To Constant12/1 -> Read_Gyro12/Trigger
  Compare To Constant11/1 -> Read_Gyro11/Trigger
  Compare To Constant10/1 -> Read_Gyro10/Trigger
  Compare To Constant5/1 -> Read_Gyro5/Trigger
  Compare To Constant7/1 -> Read_Gyro7/Trigger
  Compare To Constant3/1 -> Read_Gyro3/Trigger
  Read_Gyro2/1(Out1) -> Terminator2/1
  Read_Gyro3/1(Out1) -> Terminator3/1
  Compare To Constant9/1 -> Read_Gyro9/Trigger
  Compare To Constant6/1 -> Read_Gyro6/Trigger
  Compare To Constant4/1 -> Read_Gyro4/Trigger
  Compare To Constant/1 -> Read_Gyro/Trigger
  Read_Gyro/1(Out1) -> Terminator/1
  Compare To Constant1/1 -> Read_Gyro1/Trigger
  Compare To Constant2/1 -> Read_Gyro2/Trigger
  Read_Gyro1/1(Out1) -> check/1  "Check_ID2_Current2"
  Read_Gyro16/1(Out1) -> Terminator1/1
  Read_Gyro4/1(Out1) -> Bus Creator/1
  Read_Gyro5/1(Out1) -> Bus Creator/2
  Read_Gyro7/1(Out1) -> Bus Creator/4
  Read_Gyro6/1(Out1) -> Bus Creator/3
  Bus Creator/1 -> byte1/1
  Bus Creator1/1 -> byte6/1
  Read_Gyro8/1(Out1) -> Bus Creator1/1
  Read_Gyro9/1(Out1) -> Bus Creator1/2
  Read_Gyro10/1(Out1) -> Bus Creator1/3
  Read_Gyro11/1(Out1) -> Bus Creator1/4
  Read_Gyro12/1(Out1) -> Bus Creator2/1
  Read_Gyro13/1(Out1) -> Bus Creator2/2
  Read_Gyro14/1(Out1) -> Bus Creator2/3
  Read_Gyro15/1(Out1) -> Bus Creator2/4
  Bus Creator2/1 -> byte12/1

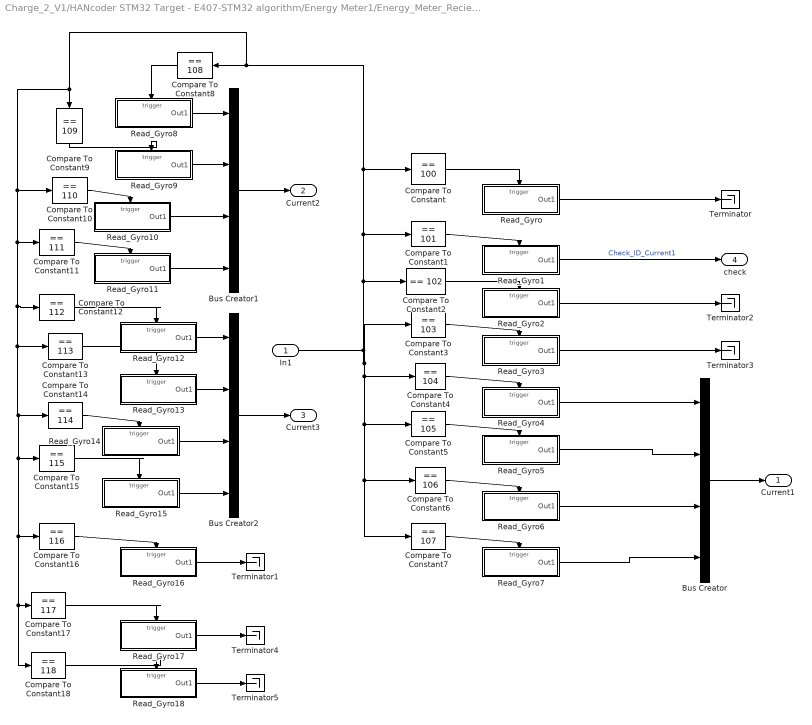
== system Charge_2_V1/HANcoder STM32 Target - E407-STM32 algorithm/Energy Meter1/Energy_Meter_Recieve/Current_Meter ==
  In1 : Inport
  Bus Creator : BusCreator  Inputs=4
  Bus Creator1 : BusCreator  Inputs=4
  Bus Creator2 : BusCreator  Inputs=4
  Compare To Constant : simulink/Logic and Bit Operations/Compare To Constant  relop===  const=100  OutDataTypeStr=uint8
  Compare To Constant1 : simulink/Logic and Bit Operations/Compare To Constant  relop===  const=101  OutDataTypeStr=uint8
  Compare To Constant10 : simulink/Logic and Bit Operations/Compare To Constant  relop===  const=110  OutDataTypeStr=uint8
  Compare To Constant11 : simulink/Logic and Bit Operations/Compare To Constant  relop===  const=111  OutDataTypeStr=uint8
  Compare To Constant12 : simulink/Logic and Bit Operations/Compare To Constant  relop===  const=112  OutDataTypeStr=uint8
  Compare To Constant13 : simulink/Logic and Bit Operations/Compare To Constant  relop===  const=113  OutDataTypeStr=uint8
  Compare To Constant14 : simulink/Logic and Bit Operations/Compare To Constant  relop===  const=114  OutDataTypeStr=uint8
  Compare To Constant15 : simulink/Logic and Bit Operations/Compare To Constant  relop===  const=115  OutDataTypeStr=uint8
  Compare To Constant16 : simulink/Logic and Bit Operations/Compare To Constant  relop===  const=116  OutDataTypeStr=uint8
  Compare To Constant17 : simulink/Logic and Bit Operations/Compare To Constant  relop===  const=117  OutDataTypeStr=uint8
  Compare To Constant18 : simulink/Logic and Bit Operations/Compare To Constant  relop===  const=118  OutDataTypeStr=uint8
  Compare To Constant2 : simulink/Logic and Bit Operations/Compare To Constant  relop===  const=102  OutDataTypeStr=uint8
  Compare To Constant3 : simulink/Logic and Bit Operations/Compare To Constant  relop===  const=103  OutDataTypeStr=uint8
  Compare To Constant4 : simulink/Logic and Bit Operations/Compare To Constant  relop===  const=104  OutDataTypeStr=uint8
  Compare To Constant5 : simulink/Logic and Bit Operations/Compare To Constant  relop===  const=105  OutDataTypeStr=uint8
  Compare To Constant6 : simulink/Logic and Bit Operations/Compare To Constant  relop===  const=106  OutDataTypeStr=uint8
  Compare To Constant7 : simulink/Logic and Bit Operations/Compare To Constant  relop===  const=107  OutDataTypeStr=uint8
  Compare To Constant8 : simulink/Logic and Bit Operations/Compare To Constant  relop===  const=108  OutDataTypeStr=uint8
  Compare To Constant9 : simulink/Logic and Bit Operations/Compare To Constant  relop===  const=109  OutDataTypeStr=uint8
  Read_Gyro : Subsystem  TreatAsAtomicUnit=on
  Read_Gyro1 : Subsystem  TreatAsAtomicUnit=on
  Read_Gyro10 : Subsystem  TreatAsAtomicUnit=on
  Read_Gyro11 : Subsystem  TreatAsAtomicUnit=on
  Read_Gyro12 : Subsystem  TreatAsAtomicUnit=on
  Read_Gyro13 : Subsystem  TreatAsAtomicUnit=on
  Read_Gyro14 : Subsystem  TreatAsAtomicUnit=on
  Read_Gyro15 : Subsystem  TreatAsAtomicUnit=on
  Read_Gyro16 : Subsystem  TreatAsAtomicUnit=on
  Read_Gyro17 : Subsystem  TreatAsAtomicUnit=on
  Read_Gyro18 : Subsystem  TreatAsAtomicUnit=on
  Read_Gyro2 : Subsystem  TreatAsAtomicUnit=on
  Read_Gyro3 : Subsystem  TreatAsAtomicUnit=on
  Read_Gyro4 : Subsystem  TreatAsAtomicUnit=on
  Read_Gyro5 : Subsystem  TreatAsAtomicUnit=on
  Read_Gyro6 : Subsystem  TreatAsAtomicUnit=on
  Read_Gyro7 : Subsystem  TreatAsAtomicUnit=on
  Read_Gyro8 : Subsystem  TreatAsAtomicUnit=on
  Read_Gyro9 : Subsystem  TreatAsAtomicUnit=on
  Terminator{,1..5} (6 alike) : Terminator
  Current1 : Outport
  Current2 : Outport  Port=2
  Current3 : Outport  Port=3
  check : Outport  Port=4
  wires:
  Read_Gyro1/1(Out1) -> check/1  "Check_ID_Current1"
  Compare To Constant2/1 -> Read_Gyro2/Trigger
  Compare To Constant1/1 -> Read_Gyro1/Trigger
  Read_Gyro/1(Out1) -> Terminator/1
  Compare To Constant/1 -> Read_Gyro/Trigger
  Compare To Constant4/1 -> Read_Gyro4/Trigger
  Compare To Constant6/1 -> Read_Gyro6/Trigger
  Compare To Constant9/1 -> Read_Gyro9/Trigger
  Read_Gyro6/1(Out1) -> Bus Creator/3
  Read_Gyro3/1(Out1) -> Terminator3/1
  Read_Gyro2/1(Out1) -> Terminator2/1
  Compare To Constant3/1 -> Read_Gyro3/Trigger
  Compare To Constant7/1 -> Read_Gyro7/Trigger
  Compare To Constant5/1 -> Read_Gyro5/Trigger
  Compare To Constant10/1 -> Read_Gyro10/Trigger
  Read_Gyro5/1(Out1) -> Bus Creator/2
  Read_Gyro7/1(Out1) -> Bus Creator/4
  Compare To Constant11/1 -> Read_Gyro11/Trigger
  Compare To Constant12/1 -> Read_Gyro12/Trigger
  Compare To Constant13/1 -> Read_Gyro13/Trigger
  In1/1 -> Compare To Constant7/1, Compare To Constant6/1, Compare To Constant5/1, Compare To Constant4/1, Compare To Constant3/1, Compare To Constant11/1, Compare To Constant12/1, Compare To Constant18/1, Compare To Constant17/1, Compare To Constant16/1, Compare To Constant15/1, Compare To Constant14/1, Compare To Constant13/1, Compare To Constant10/1, Compare To Constant9/1, Compare To Constant8/1, Compare To Constant/1, Compare To Constant1/1, Compare To Constant2/1
  Compare To Constant8/1 -> Read_Gyro8/Trigger
  Compare To Constant14/1 -> Read_Gyro14/Trigger
  Compare To Constant15/1 -> Read_Gyro15/Trigger
  Compare To Constant16/1 -> Read_Gyro16/Trigger
  Compare To Constant17/1 -> Read_Gyro17/Trigger
  Compare To Constant18/1 -> Read_Gyro18/Trigger
  Read_Gyro16/1(Out1) -> Terminator1/1
  Read_Gyro17/1(Out1) -> Terminator4/1
  Read_Gyro18/1(Out1) -> Terminator5/1
  Read_Gyro4/1(Out1) -> Bus Creator/1
  Bus Creator/1 -> Current1/1
  Read_Gyro8/1(Out1) -> Bus Creator1/1
  Read_Gyro9/1(Out1) -> Bus Creator1/2
  Read_Gyro10/1(Out1) -> Bus Creator1/3
  Read_Gyro11/1(Out1) -> Bus Creator1/4
  Bus Creator1/1 -> Current2/1
  Read_Gyro12/1(Out1) -> Bus Creator2/1
  Read_Gyro13/1(Out1) -> Bus Creator2/2
  Read_Gyro14/1(Out1) -> Bus Creator2/3
  Read_Gyro15/1(Out1) -> Bus Creator2/4
  Bus Creator2/1 -> Current3/1

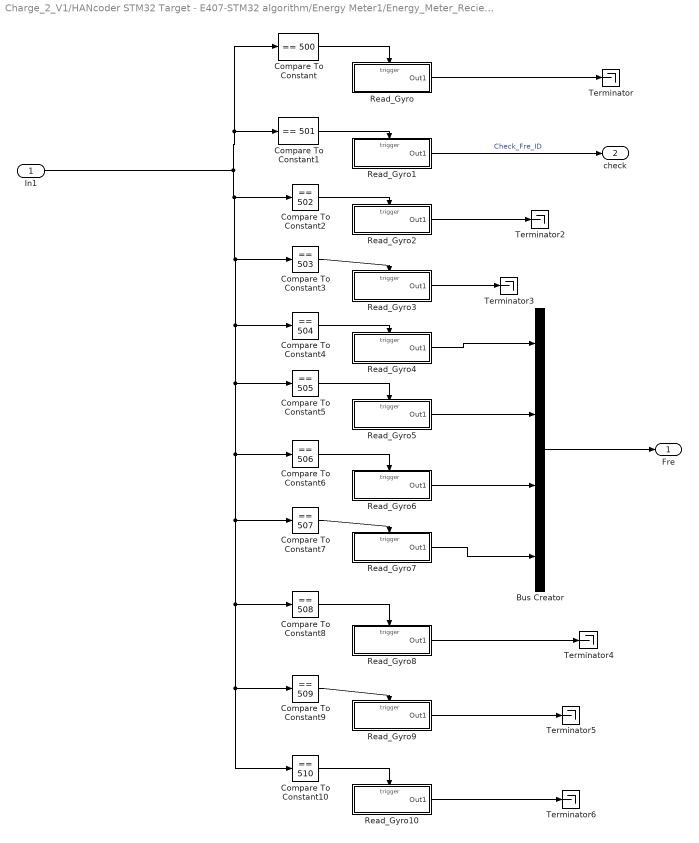
== system Charge_2_V1/HANcoder STM32 Target - E407-STM32 algorithm/Energy Meter1/Energy_Meter_Recieve/Fequency ==
  In1 : Inport
  Bus Creator : BusCreator  Inputs=4
  Compare To Constant : simulink/Logic and Bit Operations/Compare To Constant  relop===  const=500  OutDataTypeStr=uint8
  Compare To Constant1 : simulink/Logic and Bit Operations/Compare To Constant  relop===  const=501  OutDataTypeStr=uint8
  Compare To Constant10 : simulink/Logic and Bit Operations/Compare To Constant  relop===  const=510  OutDataTypeStr=uint8
  Compare To Constant2 : simulink/Logic and Bit Operations/Compare To Constant  relop===  const=502  OutDataTypeStr=uint8
  Compare To Constant3 : simulink/Logic and Bit Operations/Compare To Constant  relop===  const=503  OutDataTypeStr=uint8
  Compare To Constant4 : simulink/Logic and Bit Operations/Compare To Constant  relop===  const=504  OutDataTypeStr=uint8
  Compare To Constant5 : simulink/Logic and Bit Operations/Compare To Constant  relop===  const=505  OutDataTypeStr=uint8
  Compare To Constant6 : simulink/Logic and Bit Operations/Compare To Constant  relop===  const=506  OutDataTypeStr=uint8
  Compare To Constant7 : simulink/Logic and Bit Operations/Compare To Constant  relop===  const=507  OutDataTypeStr=uint8
  Compare To Constant8 : simulink/Logic and Bit Operations/Compare To Constant  relop===  const=508  OutDataTypeStr=uint8
  Compare To Constant9 : simulink/Logic and Bit Operations/Compare To Constant  relop===  const=509  OutDataTypeStr=uint8
  Read_Gyro : Subsystem  TreatAsAtomicUnit=on
  Read_Gyro1 : Subsystem  TreatAsAtomicUnit=on
  Read_Gyro10 : Subsystem  TreatAsAtomicUnit=on
  Read_Gyro2 : Subsystem  TreatAsAtomicUnit=on
  Read_Gyro3 : Subsystem  TreatAsAtomicUnit=on
  Read_Gyro4 : Subsystem  TreatAsAtomicUnit=on
  Read_Gyro5 : Subsystem  TreatAsAtomicUnit=on
  Read_Gyro6 : Subsystem  TreatAsAtomicUnit=on
  Read_Gyro7 : Subsystem  TreatAsAtomicUnit=on
  Read_Gyro8 : Subsystem  TreatAsAtomicUnit=on
  Read_Gyro9 : Subsystem  TreatAsAtomicUnit=on
  Terminator{,2..6} (6 alike) : Terminator
  Fre : Outport
  check : Outport  Port=2
  wires:
  Read_Gyro1/1(Out1) -> check/1  "Check_Fre_ID"
  Compare To Constant2/1 -> Read_Gyro2/Trigger
  Compare To Constant1/1 -> Read_Gyro1/Trigger
  In1/1 -> Compare To Constant/1, Compare To Constant1/1, Compare To Constant10/1, Compare To Constant9/1, Compare To Constant8/1, Compare To Constant7/1, Compare To Constant6/1, Compare To Constant5/1, Compare To Constant4/1, Compare To Constant3/1, Compare To Constant2/1
  Read_Gyro/1(Out1) -> Terminator/1
  Compare To Constant/1 -> Read_Gyro/Trigger
  Read_Gyro8/1(Out1) -> Terminator4/1
  Compare To Constant4/1 -> Read_Gyro4/Trigger
  Compare To Constant6/1 -> Read_Gyro6/Trigger
  Compare To Constant8/1 -> Read_Gyro8/Trigger
  Compare To Constant9/1 -> Read_Gyro9/Trigger
  Compare To Constant3/1 -> Read_Gyro3/Trigger
  Compare To Constant7/1 -> Read_Gyro7/Trigger
  Compare To Constant5/1 -> Read_Gyro5/Trigger
  Compare To Constant10/1 -> Read_Gyro10/Trigger
  Read_Gyro10/1(Out1) -> Terminator6/1
  Read_Gyro9/1(Out1) -> Terminator5/1
  Read_Gyro2/1(Out1) -> Terminator2/1
  Read_Gyro3/1(Out1) -> Terminator3/1
  Read_Gyro4/1(Out1) -> Bus Creator/1
  Read_Gyro5/1(Out1) -> Bus Creator/2
  Read_Gyro6/1(Out1) -> Bus Creator/3
  Read_Gyro7/1(Out1) -> Bus Creator/4
  Bus Creator/1 -> Fre/1
